simulink model "Copy_of_VTOLTiltrotor"  (R2024a)
settings: configuration reference "VTOLConfiguration" (kept outside this file)
undefined symbols (not defined in the file): airspeed, Battery, BCE12, BCE_Set_init, BMS_Controller_State, C, Cell10_P, Cell11_P, Cell12_P, Cell1_N, Cell1_P, Cell2_P, Cell3_P, Cell4_P, Cell5_P, Cell6_P, Cell7_P, Cell8_P, Cell9_P, Cell_Temperatures, Cell_Voltages, Charging_State, CityMission, control, controlParams, ControlSampleTime, CriticalTiltAngle, currentFactor, CV_Gain, ddx, ddy, ddz, Device_01, DiscIntNeverNeededParam, dx, dy, dz, Earth, env, F, F28379D_ADC_MaxCount, F28379D_ADC_Vmax, FixedWingMission, flightState, Foc_Ki_IxTcpu, Foc_Ki_S, Foc_Kp_I, Foc_Kp_S, fractalcoef, FSState, FWControlParams, HoverMission, I_cc, Ia_offset, Ib_offset, iniRoll, initPitch, iniYaw, IO334, IO334_DAC_Vmax ... (+55)
libraries: slrealtimeethercatlib x109, simulink x81, fl_lib x65, slpidlib x49, mcbcontrolslib x48, nesl_utility x43, speedgoatlib_hdlCoder_IO3xx x31, canmsglib x17, slrealtimeutilitieslib x13, mcbhdlplantlib x13, speedgoatlib_IO611 x12, dspstat3 x12
(part 11 of 20)

== system Copy_of_VTOLTiltrotor/Flight Controller/Autopilot/Multicopter Controller/Horizontal Position Control/XY Controller ==
  X_ref : Inport
  Y_ref : Inport  Port=2
  States : Inport  Port=3
  Bus Selector : BusSelector  OutputSignals=Xe,Ve,Euler
  Demux : Demux  Outputs=3
  Demux1 : Demux  Outputs=3
  Demux2 : Demux  Outputs=3
  Gain : Gain
  Saturation : Saturate  UpperLimit=5  LowerLimit=-5
  Saturation1 : Saturate  UpperLimit=5  LowerLimit=-5
  Sum{,1..3} (4 alike) : Sum  Inputs=|+-
  Terminator{,1..3} (4 alike) : Terminator
  Vx Controller : slpidlib/PID Controller  Controller=P  Form=Parallel  TimeDomain=Discrete-time  UseExternalTs=off  SampleTime=0.005  IntegratorMethod=Forward Euler  FilterMethod=Forward Euler  ControllerParametersSource=internal  P=controlParams.P_VX  I=0  UseKiTs=off  D=0.0379422021775223  UseExternalDerivativeSource=off  N=1.96946409823213  UseFilter=on  TunerSelectOption=Transfer Function Based (PID Tuner App)  InitialConditionSource=internal  InitialConditionForIntegrator=0  InitialConditionForFilter=0  DifferentiatorICPrevScaledInput=0  ExternalReset=none  TrackingMode=off  Kt=1  LimitOutput=off  SatLimitsSource=internal  UpperSaturationLimit=inf  LowerSaturationLimit=-inf  LinearizeAsGain=on  AntiWindupMode=none  Kb=1  LimitIntegrator=off  UpperIntegratorSaturationLimit=inf  LowerIntegratorSaturationLimit=-inf  POutMin=[]  POutMax=[]  IOutMin=[]  IOutMax=[]  DOutMin=[]  DOutMax=[]  NOutMin=[]  NOutMax=[]  SumOutMin=[]  SumOutMax=[]  SaturationOutMin=[]  SaturationOutMax=[]  PParamMin=[]  PParamMax=[]  IParamMin=[]  IParamMax=[]  DParamMin=[]  DParamMax=[]  NParamMin=[]  NParamMax=[]  KbParamMin=[]  KbParamMax=[]  KtParamMin=[]  KtParamMax=[]  KbOutMin=[]  KbOutMax=[]  KtOutMin=[]  KtOutMax=[]  IntegratorOutMin=[]  IntegratorOutMax=[]  FilterOutMin=[]  FilterOutMax=[]  SumI1OutMin=[]  SumI1OutMax=[]  SumI2OutMin=[]  SumI2OutMax=[]  SumI3OutMin=[]  SumI3OutMax=[]  SumI4OutMin=[]  SumI4OutMax=[]  SumDOutMin=[]  SumDOutMax=[]  DifferentiatorOutMin=[]  DifferentiatorOutMax=[]  FilterDiffOutCoefMin=[]  FilterDiffOutCoefMax=[]  ReciprocalOutMin=[]  ReciprocalOutMax=[]  SumDenOutMin=[]  SumDenOutMax=[]  SumNumOutMin=[]  SumNumOutMax=[]  DivideOutMin=[]  DivideOutMax=[]  UdiffTsProdOutMin=[]  UdiffTsProdOutMax=[]  NTsProdOutMin=[]  NTsProdOutMax=[]  UintegralTsProdOutMin=[]  UintegralTsProdOutMax=[]  UngainTsProdOutMin=[]  UngainTsProdOutMax=[]  ClampingZeroOutDataTypeStr=Inherit: Inherit via back propagation  ClampingZeroOutMin=[]  ClampingZeroOutMax=[]  FilterDenConstantOutDataTypeStr=Inherit: Inherit via back propagation  FilterDenConstantOutMin=[]  FilterDenConstantOutMax=[]  PCopyOutDataTypeStr=Inherit: Inherit via back propagation  PCopyOutMin=[]  PCopyOutMax=[]  NCopyOutDataTypeStr=Inherit: Inherit via back propagation  NCopyOutMin=[]  NCopyOutMax=[]  IntegratorContinuousStateAttributes=''  IntegratorStateMustResolveToSignalObject=off  IntegratorRTWStateStorageClass=Auto  FilterContinuousStateAttributes=''  FilterStateMustResolveToSignalObject=off  FilterRTWStateStorageClass=Auto  ParallelPVariant=InternalParameters  IdealPVariant=Disabled  IVariant=Disabled  DVariant=Disabled  IntegratorVariant=Disabled  SatVariant=Disabled  AWVariant=Disabled  PCopyVariant=Disabled  TRVariant=Disabled  FdbkBlocksVariant=Forward  IdealPFdbkVariant=Disabled  SatFdbkVariant=Disabled  DerivativeFilterVariant=Disabled  NVariant=Disabled  NCopyVariant=Disabled_SignalSpec  FilterICVariant=Disabled  IntegratorICVariant=Disabled  ExternalResetVariant=Disabled  TRSumVariant=Passthrough  SumFdbkVariant=Disabled  SumVariant=Passthrough_P  TsampFilterVariant=InternalTs  TsampNgainVariant=Passthrough  TsampIntegralVariant=Disabled_SignalSpec  ExternalSaturationOutDataTypeStr=Inherit: Same as second input  DerivativeSourceVariant=Disabled
  Vy Controller : slpidlib/PID Controller  Controller=P  Form=Parallel  TimeDomain=Discrete-time  UseExternalTs=off  SampleTime=0.005  IntegratorMethod=Forward Euler  FilterMethod=Forward Euler  ControllerParametersSource=internal  P=controlParams.P_VY  I=0  UseKiTs=off  D=0.0379422021775223  UseExternalDerivativeSource=off  N=1.96946409823213  UseFilter=on  TunerSelectOption=Transfer Function Based (PID Tuner App)  InitialConditionSource=internal  InitialConditionForIntegrator=0  InitialConditionForFilter=0  DifferentiatorICPrevScaledInput=0  ExternalReset=none  TrackingMode=off  Kt=1  LimitOutput=off  SatLimitsSource=internal  UpperSaturationLimit=inf  LowerSaturationLimit=-inf  LinearizeAsGain=on  AntiWindupMode=none  Kb=1  LimitIntegrator=off  UpperIntegratorSaturationLimit=inf  LowerIntegratorSaturationLimit=-inf  RndMeth=Round  POutMin=[]  POutMax=[]  IOutMin=[]  IOutMax=[]  DOutMin=[]  DOutMax=[]  NOutMin=[]  NOutMax=[]  SumOutMin=[]  SumOutMax=[]  SaturationOutMin=[]  SaturationOutMax=[]  PParamMin=[]  PParamMax=[]  IParamMin=[]  IParamMax=[]  DParamMin=[]  DParamMax=[]  NParamMin=[]  NParamMax=[]  KbParamMin=[]  KbParamMax=[]  KtParamMin=[]  KtParamMax=[]  KbOutMin=[]  KbOutMax=[]  KtOutMin=[]  KtOutMax=[]  IntegratorOutMin=[]  IntegratorOutMax=[]  FilterOutMin=[]  FilterOutMax=[]  SumI1OutMin=[]  SumI1OutMax=[]  SumI2OutMin=[]  SumI2OutMax=[]  SumI3OutMin=[]  SumI3OutMax=[]  SumI4OutMin=[]  SumI4OutMax=[]  SumDOutMin=[]  SumDOutMax=[]  DifferentiatorOutMin=[]  DifferentiatorOutMax=[]  FilterDiffOutCoefMin=[]  FilterDiffOutCoefMax=[]  ReciprocalOutMin=[]  ReciprocalOutMax=[]  SumDenOutMin=[]  SumDenOutMax=[]  SumNumOutMin=[]  SumNumOutMax=[]  DivideOutMin=[]  DivideOutMax=[]  UdiffTsProdOutMin=[]  UdiffTsProdOutMax=[]  NTsProdOutMin=[]  NTsProdOutMax=[]  UintegralTsProdOutMin=[]  UintegralTsProdOutMax=[]  UngainTsProdOutMin=[]  UngainTsProdOutMax=[]  ClampingZeroOutDataTypeStr=Inherit: Inherit via back propagation  ClampingZeroOutMin=[]  ClampingZeroOutMax=[]  FilterDenConstantOutDataTypeStr=Inherit: Inherit via back propagation  FilterDenConstantOutMin=[]  FilterDenConstantOutMax=[]  PCopyOutDataTypeStr=Inherit: Inherit via back propagation  PCopyOutMin=[]  PCopyOutMax=[]  NCopyOutDataTypeStr=Inherit: Inherit via back propagation  NCopyOutMin=[]  NCopyOutMax=[]  IntegratorContinuousStateAttributes=''  IntegratorStateMustResolveToSignalObject=off  IntegratorRTWStateStorageClass=Auto  FilterContinuousStateAttributes=''  FilterStateMustResolveToSignalObject=off  FilterRTWStateStorageClass=Auto  ParallelPVariant=InternalParameters  IdealPVariant=Disabled  IVariant=Disabled  DVariant=Disabled  IntegratorVariant=Disabled  SatVariant=Disabled  AWVariant=Disabled  PCopyVariant=Disabled  TRVariant=Disabled  FdbkBlocksVariant=Forward  IdealPFdbkVariant=Disabled  SatFdbkVariant=Disabled  DerivativeFilterVariant=Disabled  NVariant=Disabled  NCopyVariant=Disabled_SignalSpec  FilterICVariant=Disabled  IntegratorICVariant=Disabled  ExternalResetVariant=Disabled  TRSumVariant=Passthrough  SumFdbkVariant=Disabled  SumVariant=Passthrough_P  TsampFilterVariant=InternalTs  TsampNgainVariant=Passthrough  TsampIntegralVariant=Disabled_SignalSpec  ExternalSaturationOutDataTypeStr=Inherit: Same as second input  DerivativeSourceVariant=Disabled
  X Controller : slpidlib/PID Controller  Controller=PID  Form=Parallel  TimeDomain=Discrete-time  UseExternalTs=off  SampleTime=-1  IntegratorMethod=Forward Euler  FilterMethod=Forward Euler  ControllerParametersSource=internal  P=controlParams.P_X  I=controlParams.I_X  UseKiTs=off  D=controlParams.D_X  UseExternalDerivativeSource=off  N=controlParams.N_X  UseFilter=on  TunerSelectOption=Transfer Function Based (PID Tuner App)  InitialConditionSource=internal  InitialConditionForIntegrator=0  InitialConditionForFilter=0  DifferentiatorICPrevScaledInput=0  ExternalReset=none  TrackingMode=off  Kt=1  LimitOutput=off  SatLimitsSource=internal  UpperSaturationLimit=inf  LowerSaturationLimit=-inf  LinearizeAsGain=on  AntiWindupMode=none  Kb=1  LimitIntegrator=off  UpperIntegratorSaturationLimit=inf  LowerIntegratorSaturationLimit=-inf  POutMin=[]  POutMax=[]  IOutMin=[]  IOutMax=[]  DOutMin=[]  DOutMax=[]  NOutMin=[]  NOutMax=[]  SumOutMin=[]  SumOutMax=[]  SaturationOutMin=[]  SaturationOutMax=[]  PParamMin=[]  PParamMax=[]  IParamMin=[]  IParamMax=[]  DParamMin=[]  DParamMax=[]  NParamMin=[]  NParamMax=[]  KbParamMin=[]  KbParamMax=[]  KtParamMin=[]  KtParamMax=[]  KbOutMin=[]  KbOutMax=[]  KtOutMin=[]  KtOutMax=[]  IntegratorOutMin=[]  IntegratorOutMax=[]  FilterOutMin=[]  FilterOutMax=[]  SumI1OutMin=[]  SumI1OutMax=[]  SumI2OutMin=[]  SumI2OutMax=[]  SumI3OutMin=[]  SumI3OutMax=[]  SumI4OutMin=[]  SumI4OutMax=[]  SumDOutMin=[]  SumDOutMax=[]  DifferentiatorOutMin=[]  DifferentiatorOutMax=[]  FilterDiffOutCoefMin=[]  FilterDiffOutCoefMax=[]  ReciprocalOutMin=[]  ReciprocalOutMax=[]  SumDenOutMin=[]  SumDenOutMax=[]  SumNumOutMin=[]  SumNumOutMax=[]  DivideOutMin=[]  DivideOutMax=[]  UdiffTsProdOutMin=[]  UdiffTsProdOutMax=[]  NTsProdOutMin=[]  NTsProdOutMax=[]  UintegralTsProdOutMin=[]  UintegralTsProdOutMax=[]  UngainTsProdOutMin=[]  UngainTsProdOutMax=[]  ClampingZeroOutDataTypeStr=Inherit: Inherit via back propagation  ClampingZeroOutMin=[]  ClampingZeroOutMax=[]  FilterDenConstantOutDataTypeStr=Inherit: Inherit via back propagation  FilterDenConstantOutMin=[]  FilterDenConstantOutMax=[]  PCopyOutDataTypeStr=Inherit: Inherit via back propagation  PCopyOutMin=[]  PCopyOutMax=[]  NCopyOutDataTypeStr=Inherit: Inherit via back propagation  NCopyOutMin=[]  NCopyOutMax=[]  IntegratorContinuousStateAttributes=''  IntegratorStateMustResolveToSignalObject=off  IntegratorRTWStateStorageClass=Auto  FilterContinuousStateAttributes=''  FilterStateMustResolveToSignalObject=off  FilterRTWStateStorageClass=Auto  ParallelPVariant=InternalParameters  IdealPVariant=Disabled  IVariant=InternalParameters  DVariant=InternalParameters  IntegratorVariant=Discrete  SatVariant=Disabled  AWVariant=Passthrough  PCopyVariant=Disabled  TRVariant=Disabled  FdbkBlocksVariant=Forward  IdealPFdbkVariant=Disabled  SatFdbkVariant=Disabled  DerivativeFilterVariant=ForwardEulerFilter  NVariant=InternalParameters  NCopyVariant=Disabled  FilterICVariant=InternalICsFilter  IntegratorICVariant=InternalICs  ExternalResetVariant=Disabled  TRSumVariant=Passthrough  SumFdbkVariant=Disabled  SumVariant=Sum_PID  TsampFilterVariant=InternalTs  TsampNgainVariant=Passthrough  TsampIntegralVariant=Disabled_SignalSpec  ExternalSaturationOutDataTypeStr=Inherit: Same as second input  DerivativeSourceVariant=ErrorSignal
  Y Controller : slpidlib/PID Controller  Controller=PI  Form=Parallel  TimeDomain=Discrete-time  UseExternalTs=off  SampleTime=-1  IntegratorMethod=Forward Euler  FilterMethod=Forward Euler  ControllerParametersSource=internal  P=controlParams.P_Y  I=controlParams.I_Y  UseKiTs=off  D=controlParams.D_Y/10  UseExternalDerivativeSource=off  N=controlParams.N_Y  UseFilter=on  TunerSelectOption=Transfer Function Based (PID Tuner App)  InitialConditionSource=internal  InitialConditionForIntegrator=0  InitialConditionForFilter=0  DifferentiatorICPrevScaledInput=0  ExternalReset=none  TrackingMode=off  Kt=1  LimitOutput=off  SatLimitsSource=internal  UpperSaturationLimit=0.4  LowerSaturationLimit=-0.4  LinearizeAsGain=on  AntiWindupMode=clamping  Kb=1  LimitIntegrator=off  UpperIntegratorSaturationLimit=inf  LowerIntegratorSaturationLimit=-inf  POutMin=[]  POutMax=[]  IOutMin=[]  IOutMax=[]  DOutMin=[]  DOutMax=[]  NOutMin=[]  NOutMax=[]  SumOutMin=[]  SumOutMax=[]  SaturationOutMin=[]  SaturationOutMax=[]  PParamMin=[]  PParamMax=[]  IParamMin=[]  IParamMax=[]  DParamMin=[]  DParamMax=[]  NParamMin=[]  NParamMax=[]  KbParamMin=[]  KbParamMax=[]  KtParamMin=[]  KtParamMax=[]  KbOutMin=[]  KbOutMax=[]  KtOutMin=[]  KtOutMax=[]  IntegratorOutMin=[]  IntegratorOutMax=[]  FilterOutMin=[]  FilterOutMax=[]  SumI1OutMin=[]  SumI1OutMax=[]  SumI2OutMin=[]  SumI2OutMax=[]  SumI3OutMin=[]  SumI3OutMax=[]  SumI4OutMin=[]  SumI4OutMax=[]  SumDOutMin=[]  SumDOutMax=[]  DifferentiatorOutMin=[]  DifferentiatorOutMax=[]  FilterDiffOutCoefMin=[]  FilterDiffOutCoefMax=[]  ReciprocalOutMin=[]  ReciprocalOutMax=[]  SumDenOutMin=[]  SumDenOutMax=[]  SumNumOutMin=[]  SumNumOutMax=[]  DivideOutMin=[]  DivideOutMax=[]  UdiffTsProdOutMin=[]  UdiffTsProdOutMax=[]  NTsProdOutMin=[]  NTsProdOutMax=[]  UintegralTsProdOutMin=[]  UintegralTsProdOutMax=[]  UngainTsProdOutMin=[]  UngainTsProdOutMax=[]  ClampingZeroOutDataTypeStr=Inherit: Inherit via back propagation  ClampingZeroOutMin=[]  ClampingZeroOutMax=[]  FilterDenConstantOutDataTypeStr=Inherit: Inherit via back propagation  FilterDenConstantOutMin=[]  FilterDenConstantOutMax=[]  PCopyOutDataTypeStr=Inherit: Inherit via back propagation  PCopyOutMin=[]  PCopyOutMax=[]  NCopyOutDataTypeStr=Inherit: Inherit via back propagation  NCopyOutMin=[]  NCopyOutMax=[]  IntegratorContinuousStateAttributes=''  IntegratorStateMustResolveToSignalObject=off  IntegratorRTWStateStorageClass=Auto  FilterContinuousStateAttributes=''  FilterStateMustResolveToSignalObject=off  FilterRTWStateStorageClass=Auto  ParallelPVariant=InternalParameters  IdealPVariant=Disabled  IVariant=InternalParameters  DVariant=Disabled  IntegratorVariant=Discrete  SatVariant=Disabled  AWVariant=Passthrough  PCopyVariant=Disabled  TRVariant=Disabled  FdbkBlocksVariant=Forward  IdealPFdbkVariant=Disabled  SatFdbkVariant=Disabled  DerivativeFilterVariant=Disabled  NVariant=Disabled  NCopyVariant=Disabled_SignalSpec  FilterICVariant=Disabled  IntegratorICVariant=InternalICs  ExternalResetVariant=Disabled  TRSumVariant=Passthrough  SumFdbkVariant=Disabled  SumVariant=Sum_PI  TsampFilterVariant=InternalTs  TsampNgainVariant=Passthrough  TsampIntegralVariant=Disabled_SignalSpec  ExternalSaturationOutDataTypeStr=Inherit: Same as second input  DerivativeSourceVariant=Disabled
  Yaw Correction : MATLAB Function  TreatAsAtomicUnit=on
  Forward cmd : Outport
  Sideward Cmd : Outport  Port=2
  wires:
  Sum/1 -> X Controller/1
  Demux/3 -> Terminator/1
  Demux2/3 -> Yaw Correction/3(yaw)
  Yaw Correction/1(ucmd) -> Forward cmd/1
  Bus Selector/3 -> Demux2/1  "<Euler>"
  Demux1/1 -> Sum2/2
  Demux/1 -> Sum/2
  Demux/2 -> Sum1/2
  Demux2/2 -> Terminator3/1
  Demux2/1 -> Terminator2/1
  Sum1/1 -> Y Controller/1
  Sum2/1 -> Vx Controller/1
  Yaw Correction/2(vcmd) -> Sideward Cmd/1
  Demux1/3 -> Terminator1/1
  States/1 -> Bus Selector/1
  Bus Selector/1 -> Demux/1  "<Xe>"
  Bus Selector/2 -> Demux1/1  "<Ve>"
  Vx Controller/1 -> Yaw Correction/1(xcmd)
  Demux1/2 -> Gain/1
  Sum3/1 -> Vy Controller/1
  Gain/1 -> Sum3/2
  Vy Controller/1 -> Yaw Correction/2(ycmd)
  Saturation/1 -> Sum3/1
  Saturation1/1 -> Sum2/1
  Y_ref/1 -> Sum1/1
  X_ref/1 -> Sum/1
  X Controller/1 -> Saturation1/1
  Y Controller/1 -> Saturation/1

== system Copy_of_VTOLTiltrotor/Flight Controller/Autopilot/Multicopter Controller/Subsystem/Triggered Subsystem ==
  YawHold : Inport
  Trigger : TriggerPort  VariantControl=(inherit)
  Reference : Outport
  wires:
  YawHold/1 -> Reference/1

== system Copy_of_VTOLTiltrotor/Flight Controller/Guidance Test Bench/ControlType/Guidance Testbench/Control Rate Transition ==
  "1 " : Inport
  In2 : Inport  Port=2
  In3 : Inport  Port=3
  In4 : Inport  Port=4
  In5 : Inport  Port=5
  Rate Transition{,1..3} (4 alike) : RateTransition  OutPortSampleTime=ControlSampleTime
  Rate Transition4 : RateTransition  InitialCondition=flightState.Hover  OutPortSampleTime=ControlSampleTime
  Out1 : Outport
  Out2 : Outport  Port=2
  Out3 : Outport  Port=3
  Out4 : Outport  Port=4
  Out5 : Outport  Port=5
  wires:
  In4/1 -> Rate Transition3/1
  In2/1 -> Rate Transition1/1
  Rate Transition4/1 -> Out5/1
  In5/1 -> Rate Transition4/1
  Rate Transition3/1 -> Out4/1
  "1 "/1 -> Rate Transition/1
  Rate Transition1/1 -> Out2/1
  In3/1 -> Rate Transition2/1
  Rate Transition2/1 -> Out3/1
  Rate Transition/1 -> Out1/1

== system Copy_of_VTOLTiltrotor/Flight Controller/Guidance Test Bench/ControlType/Guidance Testbench/Guidance Logic ==
  UAVState : Inport
  GCSCommands : Inport  Port=2
  Atan2 : Trigonometry  Operator=atan2
  Bus Creator : BusCreator  Inputs=4
  Bus Selector1 : BusSelector  OutputSignals=x,y,z,vy,vx
  Demux : Demux
  Guidance Stateflow : Subsystem
  Interface : Subsystem
  Mux : Mux
  Mux2 : Mux  Inputs=2
  Subsystem : Subsystem
  HoverGuidance : Outport
  FixedWingSP : Outport  Port=2
  AACSP : Outport  Port=3
  ctrlMode : Outport  Port=4
  FlightMode : Outport  Port=5
  wires:
  Mux/1 -> Guidance Stateflow/1(Pose)
  Bus Selector1/5 -> Atan2/2  "<vx>"
  GCSCommands/1 -> Guidance Stateflow/2(GCSCommands)
  Bus Selector1/4 -> Atan2/1  "<vy>"
  Bus Selector1/3 -> Mux2/2, Mux/3  "<z>"
  Bus Selector1/2 -> Mux/2  "<y>"
  UAVState/1 -> Subsystem/1(UAVState), Interface/1(UAVState)
  Bus Selector1/1 -> Mux/1  "<x>"
  Guidance Stateflow/1(HoverCommands) -> Demux/1
  Interface/1(States) -> Bus Selector1/1
  Demux/3 -> Bus Creator/3  "Z"
  Demux/1 -> Bus Creator/1  "X"
  Demux/2 -> Bus Creator/2  "Y"
  Mux2/1 -> Guidance Stateflow/3(LandingStates)
  Atan2/1 -> Mux2/1, Mux/4
  Subsystem/1(States) -> Guidance Stateflow/4(States)
  Guidance Stateflow/3(FixedWingSP) -> FixedWingSP/1
  Guidance Stateflow/2(AACSP) -> AACSP/1
  Guidance Stateflow/4(ctrlMode) -> ctrlMode/1
  Guidance Stateflow/5(FlightMode) -> FlightMode/1
  Bus Creator/1 -> HoverGuidance/1
  Demux/4 -> Bus Creator/4  "Yaw"

== system Copy_of_VTOLTiltrotor/Flight Controller/Guidance Test Bench/ControlType/Manual Control/Command Interface ==
  note: Limit rate for Manual control to keep Flight in operational envelope
  Global Mission : Inport
  Aircraft States : Inport  Port=2
  Airspeed : Constant  Value=16
  Altitude : Constant  Value=1.781376518218607
  Basic Control  Switching : Stateflow chart  TreatAsAtomicUnit=on
  Bus Creator : BusCreator  Inputs=5  OutDataTypeStr=Bus: AAC
  Bus Creator1 : BusCreator  Inputs=4  OutDataTypeStr=Bus: FixedWingCommandBus
  Bus Creator2 : BusCreator  Inputs=4
  Constant{,1..2,5..6} (5 alike) : Constant  Value=0
  Constant4 : Constant  Value=25
  Control Rate Transition : Subsystem
  Course : Constant  Value=0
  Data Type Conversion : DataTypeConversion  OutDataTypeStr=Enum: flightState  SaturateOnIntegerOverflow=off  RndMeth=Floor
  Degrees to Radians : simulink_extras/Transformations/Degrees to Radians
  FlightModeSlider : Constant  Value=0  OutDataTypeStr=uint8
  Gain : Gain  Gain=-1
  Rate Limiter : RateLimiter  RisingSlewLimit=3  FallingSlewLimit=-3  SampleTimeMode=inherited
  Subsystem : Subsystem
  Terminator1 : Terminator
  X : Constant  Value=30
  Y : Constant  Value=30
  Z : Constant  Value=50
  ctrlMode : Outport
  FixedWingSP : Outport  Port=2
  AACSP : Outport  Port=3
  PositionCmds : Outport  Port=4
  FlightMode : Outport  Port=5
  wires:
  Global Mission/1 -> Terminator1/1
  Altitude/1 -> Bus Creator/2  "altitude"
  Bus Creator2/1 -> Control Rate Transition/5(Position)
  Constant5/1 -> Bus Creator/5  "climbrate"
  Course/1 -> Degrees to Radians/1
  Bus Creator/1 -> Control Rate Transition/4(AACSetpoint)
  Z/1 -> Gain/1  "Z"
  Data Type Conversion/1 -> Control Rate Transition/1(FM), Basic Control  Switching/1(FlightMode)
  Constant/1 -> Bus Creator1/1  "roll"
  Bus Creator1/1 -> Control Rate Transition/3(FixedWingSetpoint)
  Constant1/1 -> Bus Creator1/2  "pitch"
  Constant4/1 -> Bus Creator/4  "L1"
  Constant2/1 -> Bus Creator1/3  "yaw"
  Airspeed/1 -> Bus Creator1/4, Bus Creator/1  "airspeed"
  Control Rate Transition/2(FixedWingSP) -> FixedWingSP/1
  Degrees to Radians/1 -> Bus Creator/3  "course"
  X/1 -> Bus Creator2/1  "X"
  Aircraft States/1 -> Subsystem/1(UAVState)
  Y/1 -> Bus Creator2/2  "Y"
  Gain/1 -> Rate Limiter/1  "Z"
  Basic Control  Switching/1(controlMode) -> Control Rate Transition/2("ControlMode ")
  Control Rate Transition/1(ctrlMode) -> ctrlMode/1
  Control Rate Transition/3(AACSP) -> AACSP/1
  Control Rate Transition/4(PositionCmds) -> PositionCmds/1
  Control Rate Transition/5(FlightMode) -> FlightMode/1
  FlightModeSlider/1 -> Data Type Conversion/1
  Subsystem/1(States) -> Basic Control  Switching/2(States)
  Constant6/1 -> Bus Creator2/4
  Rate Limiter/1 -> Bus Creator2/3  "Z"

== system Copy_of_VTOLTiltrotor/Motor Control/Controller/Controller_MIL/F28379D Firmware/Controller Algorithm ==
  Ia_PU : Inport
  QEP_Position_Count : Inport  Port=2
  QEP_Index_Latch : Inport  Port=3
  SpdCmd : Inport  Port=4
  Kp_S : Inport  Port=5
  Ki_S : Inport  Port=6
  EnClosedLoop : Inport  Port=7
  EnablePWM : Inport  Port=8
  Kp_i : Inport  Port=9
  Ki_ixTcpu : Inport  Port=10
  AND : Logic  IconShape=distinctive  AllPortsSameDT=off  OutDataTypeStr=boolean
  Data Type Conversion : DataTypeConversion  OutDataTypeStr=single  SaturateOnIntegerOverflow=off  RndMeth=Floor
  Demux : Demux  Outputs=2
  FOC : Subsystem
  Gain : Gain  Gain=PU_System_I_base
  Gain1 : Gain  Gain=PU_System_N_base
  Mux : Mux  Inputs=2
  Speed and Pos Decoder : Subsystem
  pmsm.PositionOffset : Constant  Value=0  SampleTime=-1
  ModWave : Outport
  PWM_Enable : Outport  Port=2
  fbk_CAN : Outport  Port=3
  wires:
  EnClosedLoop/1 -> AND/2
  Speed and Pos Decoder/1(Theta_e) -> FOC/2(Pos)
  Ia_PU/1 -> FOC/1(Iab), Gain/1
  EnablePWM/1 -> FOC/6(EnablePWM)
  Speed and Pos Decoder/3(IndexFound) -> AND/1
  AND/1 -> FOC/4(EnClosedLoop)
  pmsm.PositionOffset/1 -> Speed and Pos Decoder/3(Offset)
  Speed and Pos Decoder/2(speed) -> FOC/3(Speedfb), Gain1/1
  FOC/2(PWM_Enable) -> PWM_Enable/1
  QEP_Index_Latch/1 -> Speed and Pos Decoder/2(QEP_Index_Latch)
  FOC/1(ModWave) -> ModWave/1  "ModWave"
  Kp_S/1 -> FOC/7(Kp_S)
  Ki_S/1 -> FOC/8(Ki_S)
  SpdCmd/1 -> FOC/5(SpeedRef)
  [Speed] -> Mux/1
  [Pos] -> Mux/2
  Mux/1 -> fbk_CAN/1
  Demux/1 -> [Ia_PU]
  Demux/2 -> [Ib_PU]
  Kp_i/1 -> FOC/9(Kp_i)
  Ki_ixTcpu/1 -> FOC/10(Ki_ixTcpu)
  Gain/1 -> Demux/1
  Gain1/1 -> [Speed]
  QEP_Position_Count/1 -> Speed and Pos Decoder/1(QEP_Position_Count), Data Type Conversion/1
  Data Type Conversion/1 -> [Pos]

== system Copy_of_VTOLTiltrotor/Motor Control/Controller/Controller_MIL/F28379D Firmware/Phase_Current_Rescaling ==
  Ia_ADC : Inport
  Ib_ADC : Inport  Port=2
  IaOffset : Inport  Port=3
  IbOffset : Inport  Port=4
  ADCtoA : Gain  Gain=10/IO334_DAC_Vmax/IO334_iDAC_gain  RndMeth=Simplest  OutDataTypeStr=Inherit: Same as input
  Add : Sum  Inputs=+-
  Add Constant : Bias  Bias=-2^11*IO334_DAC_Vmax/F28379D_ADC_Vmax  SaturateOnIntegerOverflow=off
  Get ADC Voltage : Gain  Gain=F28379D_ADC_Vmax/F28379D_ADC_MaxCount  OutDataTypeStr=single  RndMeth=Simplest
  Mux : Mux  Inputs=2
  Mux1 : Mux  Inputs=2
  PU_Conversion : Gain  Gain=1/PU_System_I_base  RndMeth=Simplest  OutDataTypeStr=Inherit: Same as input
  Rate Transition : RateTransition
  Iab_meas_PU : Outport  VectorParamsAs1DForOutWhenUnconnected=off
  wires:
  Mux1/1 -> Rate Transition/1
  Ia_ADC/1 -> Mux/1
  Ib_ADC/1 -> Mux/2
  Mux/1 -> Add Constant/1
  PU_Conversion/1 -> Iab_meas_PU/1
  IaOffset/1 -> Mux1/1
  IbOffset/1 -> Mux1/2
  Add Constant/1 -> Get ADC Voltage/1
  Get ADC Voltage/1 -> ADCtoA/1  "Currents_inDACvoltages"
  Rate Transition/1 -> Add/2
  ADCtoA/1 -> Add/1  "Currents_A"
  Add/1 -> PU_Conversion/1  "Currents_no_offset"

== system Copy_of_VTOLTiltrotor/Motor Control/Controller/Controller_MIL/F28379D Firmware/Speed Conditioning ==
  Spd[rpm] : Inport
  hz2pu : Gain  Gain=60/(PU_System_N_base *Maxon_645604_Np)  RndMeth=Simplest  OutDataTypeStr=Inherit: Same as input
  rads2hz : Gain  Gain=Maxon_645604_Np/(2*pi)
  rmp2rads : Gain  Gain=2*pi/60
  Spd[PU] : Outport
  wires:
  Spd[rpm]/1 -> rmp2rads/1
  rmp2rads/1 -> rads2hz/1
  rads2hz/1 -> hz2pu/1
  hz2pu/1 -> Spd[PU]/1

== system Copy_of_VTOLTiltrotor/Motor Control/Controller1/Controller_MIL/F28379D Firmware/Controller Algorithm ==
  Ia_PU : Inport
  QEP_Position_Count : Inport  Port=2
  QEP_Index_Latch : Inport  Port=3
  SpdCmd : Inport  Port=4
  Kp_S : Inport  Port=5
  Ki_S : Inport  Port=6
  EnClosedLoop : Inport  Port=7
  EnablePWM : Inport  Port=8
  Kp_i : Inport  Port=9
  Ki_ixTcpu : Inport  Port=10
  AND : Logic  IconShape=distinctive  AllPortsSameDT=off  OutDataTypeStr=boolean
  Data Type Conversion : DataTypeConversion  OutDataTypeStr=single  SaturateOnIntegerOverflow=off  RndMeth=Floor
  Demux : Demux  Outputs=2
  FOC : Subsystem
  Gain : Gain  Gain=PU_System_I_base
  Gain1 : Gain  Gain=PU_System_N_base
  Mux : Mux  Inputs=2
  Speed and Pos Decoder : Subsystem
  pmsm.PositionOffset : Constant  Value=0  SampleTime=-1
  ModWave : Outport
  PWM_Enable : Outport  Port=2
  fbk_CAN : Outport  Port=3
  wires:
  EnClosedLoop/1 -> AND/2
  Speed and Pos Decoder/1(Theta_e) -> FOC/2(Pos)
  Ia_PU/1 -> FOC/1(Iab), Gain/1
  EnablePWM/1 -> FOC/6(EnablePWM)
  Speed and Pos Decoder/3(IndexFound) -> AND/1
  AND/1 -> FOC/4(EnClosedLoop)
  pmsm.PositionOffset/1 -> Speed and Pos Decoder/3(Offset)
  Speed and Pos Decoder/2(speed) -> FOC/3(Speedfb), Gain1/1
  FOC/2(PWM_Enable) -> PWM_Enable/1
  QEP_Index_Latch/1 -> Speed and Pos Decoder/2(QEP_Index_Latch)
  FOC/1(ModWave) -> ModWave/1  "ModWave"
  Kp_S/1 -> FOC/7(Kp_S)
  Ki_S/1 -> FOC/8(Ki_S)
  SpdCmd/1 -> FOC/5(SpeedRef)
  [Speed] -> Mux/1
  [Pos] -> Mux/2
  Mux/1 -> fbk_CAN/1
  Demux/1 -> [Ia_PU]
  Demux/2 -> [Ib_PU]
  Kp_i/1 -> FOC/9(Kp_i)
  Ki_ixTcpu/1 -> FOC/10(Ki_ixTcpu)
  Gain/1 -> Demux/1
  Gain1/1 -> [Speed]
  QEP_Position_Count/1 -> Speed and Pos Decoder/1(QEP_Position_Count), Data Type Conversion/1
  Data Type Conversion/1 -> [Pos]

== system Copy_of_VTOLTiltrotor/Motor Control/Controller1/Controller_MIL/F28379D Firmware/Phase_Current_Rescaling ==
  Ia_ADC : Inport
  Ib_ADC : Inport  Port=2
  IaOffset : Inport  Port=3
  IbOffset : Inport  Port=4
  ADCtoA : Gain  Gain=10/IO334_DAC_Vmax/IO334_iDAC_gain  RndMeth=Simplest  OutDataTypeStr=Inherit: Same as input
  Add : Sum  Inputs=+-
  Add Constant : Bias  Bias=-2^11*IO334_DAC_Vmax/F28379D_ADC_Vmax  SaturateOnIntegerOverflow=off
  Get ADC Voltage : Gain  Gain=F28379D_ADC_Vmax/F28379D_ADC_MaxCount  OutDataTypeStr=single  RndMeth=Simplest
  Mux : Mux  Inputs=2
  Mux1 : Mux  Inputs=2
  PU_Conversion : Gain  Gain=1/PU_System_I_base  RndMeth=Simplest  OutDataTypeStr=Inherit: Same as input
  Rate Transition : RateTransition
  Iab_meas_PU : Outport  VectorParamsAs1DForOutWhenUnconnected=off
  wires:
  Mux1/1 -> Rate Transition/1
  Ia_ADC/1 -> Mux/1
  Ib_ADC/1 -> Mux/2
  Mux/1 -> Add Constant/1
  PU_Conversion/1 -> Iab_meas_PU/1
  IaOffset/1 -> Mux1/1
  IbOffset/1 -> Mux1/2
  Add Constant/1 -> Get ADC Voltage/1
  Get ADC Voltage/1 -> ADCtoA/1  "Currents_inDACvoltages"
  Rate Transition/1 -> Add/2
  ADCtoA/1 -> Add/1  "Currents_A"
  Add/1 -> PU_Conversion/1  "Currents_no_offset"

== system Copy_of_VTOLTiltrotor/Motor Control/Controller1/Controller_MIL/F28379D Firmware/Speed Conditioning ==
  Spd[rpm] : Inport
  hz2pu : Gain  Gain=60/(PU_System_N_base *Maxon_645604_Np)  RndMeth=Simplest  OutDataTypeStr=Inherit: Same as input
  rads2hz : Gain  Gain=Maxon_645604_Np/(2*pi)
  rmp2rads : Gain  Gain=2*pi/60
  Spd[PU] : Outport
  wires:
  Spd[rpm]/1 -> rmp2rads/1
  rmp2rads/1 -> rads2hz/1
  rads2hz/1 -> hz2pu/1
  hz2pu/1 -> Spd[PU]/1

== system Copy_of_VTOLTiltrotor/Motor Control/Controller2/Controller_MIL/F28379D Firmware/Controller Algorithm ==
  Ia_PU : Inport
  QEP_Position_Count : Inport  Port=2
  QEP_Index_Latch : Inport  Port=3
  SpdCmd : Inport  Port=4
  Kp_S : Inport  Port=5
  Ki_S : Inport  Port=6
  EnClosedLoop : Inport  Port=7
  EnablePWM : Inport  Port=8
  Kp_i : Inport  Port=9
  Ki_ixTcpu : Inport  Port=10
  AND : Logic  IconShape=distinctive  AllPortsSameDT=off  OutDataTypeStr=boolean
  Data Type Conversion : DataTypeConversion  OutDataTypeStr=single  SaturateOnIntegerOverflow=off  RndMeth=Floor
  Demux : Demux  Outputs=2
  FOC : Subsystem
  Gain : Gain  Gain=PU_System_I_base
  Gain1 : Gain  Gain=PU_System_N_base
  Mux : Mux  Inputs=2
  Speed and Pos Decoder : Subsystem
  pmsm.PositionOffset : Constant  Value=0  SampleTime=-1
  ModWave : Outport
  PWM_Enable : Outport  Port=2
  fbk_CAN : Outport  Port=3
  wires:
  EnClosedLoop/1 -> AND/2
  Speed and Pos Decoder/1(Theta_e) -> FOC/2(Pos)
  Ia_PU/1 -> FOC/1(Iab), Gain/1
  EnablePWM/1 -> FOC/6(EnablePWM)
  Speed and Pos Decoder/3(IndexFound) -> AND/1
  AND/1 -> FOC/4(EnClosedLoop)
  pmsm.PositionOffset/1 -> Speed and Pos Decoder/3(Offset)
  Speed and Pos Decoder/2(speed) -> FOC/3(Speedfb), Gain1/1
  FOC/2(PWM_Enable) -> PWM_Enable/1
  QEP_Index_Latch/1 -> Speed and Pos Decoder/2(QEP_Index_Latch)
  FOC/1(ModWave) -> ModWave/1  "ModWave"
  Kp_S/1 -> FOC/7(Kp_S)
  Ki_S/1 -> FOC/8(Ki_S)
  SpdCmd/1 -> FOC/5(SpeedRef)
  [Speed] -> Mux/1
  [Pos] -> Mux/2
  Mux/1 -> fbk_CAN/1
  Demux/1 -> [Ia_PU]
  Demux/2 -> [Ib_PU]
  Kp_i/1 -> FOC/9(Kp_i)
  Ki_ixTcpu/1 -> FOC/10(Ki_ixTcpu)
  Gain/1 -> Demux/1
  Gain1/1 -> [Speed]
  QEP_Position_Count/1 -> Speed and Pos Decoder/1(QEP_Position_Count), Data Type Conversion/1
  Data Type Conversion/1 -> [Pos]

== system Copy_of_VTOLTiltrotor/Motor Control/Controller2/Controller_MIL/F28379D Firmware/Phase_Current_Rescaling ==
  Ia_ADC : Inport
  Ib_ADC : Inport  Port=2
  IaOffset : Inport  Port=3
  IbOffset : Inport  Port=4
  ADCtoA : Gain  Gain=10/IO334_DAC_Vmax/IO334_iDAC_gain  RndMeth=Simplest  OutDataTypeStr=Inherit: Same as input
  Add : Sum  Inputs=+-
  Add Constant : Bias  Bias=-2^11*IO334_DAC_Vmax/F28379D_ADC_Vmax  SaturateOnIntegerOverflow=off
  Get ADC Voltage : Gain  Gain=F28379D_ADC_Vmax/F28379D_ADC_MaxCount  OutDataTypeStr=single  RndMeth=Simplest
  Mux : Mux  Inputs=2
  Mux1 : Mux  Inputs=2
  PU_Conversion : Gain  Gain=1/PU_System_I_base  RndMeth=Simplest  OutDataTypeStr=Inherit: Same as input
  Rate Transition : RateTransition
  Iab_meas_PU : Outport  VectorParamsAs1DForOutWhenUnconnected=off
  wires:
  Mux1/1 -> Rate Transition/1
  Ia_ADC/1 -> Mux/1
  Ib_ADC/1 -> Mux/2
  Mux/1 -> Add Constant/1
  PU_Conversion/1 -> Iab_meas_PU/1
  IaOffset/1 -> Mux1/1
  IbOffset/1 -> Mux1/2
  Add Constant/1 -> Get ADC Voltage/1
  Get ADC Voltage/1 -> ADCtoA/1  "Currents_inDACvoltages"
  Rate Transition/1 -> Add/2
  ADCtoA/1 -> Add/1  "Currents_A"
  Add/1 -> PU_Conversion/1  "Currents_no_offset"

== system Copy_of_VTOLTiltrotor/Motor Control/Controller2/Controller_MIL/F28379D Firmware/Speed Conditioning ==
  Spd[rpm] : Inport
  hz2pu : Gain  Gain=60/(PU_System_N_base *Maxon_645604_Np)  RndMeth=Simplest  OutDataTypeStr=Inherit: Same as input
  rads2hz : Gain  Gain=Maxon_645604_Np/(2*pi)
  rmp2rads : Gain  Gain=2*pi/60
  Spd[PU] : Outport
  wires:
  Spd[rpm]/1 -> rmp2rads/1
  rmp2rads/1 -> rads2hz/1
  rads2hz/1 -> hz2pu/1
  hz2pu/1 -> Spd[PU]/1

== system Copy_of_VTOLTiltrotor/Motor Control/Controller3/Controller_MIL/F28379D Firmware/Controller Algorithm ==
  Ia_PU : Inport
  QEP_Position_Count : Inport  Port=2
  QEP_Index_Latch : Inport  Port=3
  SpdCmd : Inport  Port=4
  Kp_S : Inport  Port=5
  Ki_S : Inport  Port=6
  EnClosedLoop : Inport  Port=7
  EnablePWM : Inport  Port=8
  Kp_i : Inport  Port=9
  Ki_ixTcpu : Inport  Port=10
  AND : Logic  IconShape=distinctive  AllPortsSameDT=off  OutDataTypeStr=boolean
  Data Type Conversion : DataTypeConversion  OutDataTypeStr=single  SaturateOnIntegerOverflow=off  RndMeth=Floor
  Demux : Demux  Outputs=2
  FOC : Subsystem
  Gain : Gain  Gain=PU_System_I_base
  Gain1 : Gain  Gain=PU_System_N_base
  Mux : Mux  Inputs=2
  Speed and Pos Decoder : Subsystem
  pmsm.PositionOffset : Constant  Value=0  SampleTime=-1
  ModWave : Outport
  PWM_Enable : Outport  Port=2
  fbk_CAN : Outport  Port=3
  wires:
  EnClosedLoop/1 -> AND/2
  Speed and Pos Decoder/1(Theta_e) -> FOC/2(Pos)
  Ia_PU/1 -> FOC/1(Iab), Gain/1
  EnablePWM/1 -> FOC/6(EnablePWM)
  Speed and Pos Decoder/3(IndexFound) -> AND/1
  AND/1 -> FOC/4(EnClosedLoop)
  pmsm.PositionOffset/1 -> Speed and Pos Decoder/3(Offset)
  Speed and Pos Decoder/2(speed) -> FOC/3(Speedfb), Gain1/1
  FOC/2(PWM_Enable) -> PWM_Enable/1
  QEP_Index_Latch/1 -> Speed and Pos Decoder/2(QEP_Index_Latch)
  FOC/1(ModWave) -> ModWave/1  "ModWave"
  Kp_S/1 -> FOC/7(Kp_S)
  Ki_S/1 -> FOC/8(Ki_S)
  SpdCmd/1 -> FOC/5(SpeedRef)
  [Speed] -> Mux/1
  [Pos] -> Mux/2
  Mux/1 -> fbk_CAN/1
  Demux/1 -> [Ia_PU]
  Demux/2 -> [Ib_PU]
  Kp_i/1 -> FOC/9(Kp_i)
  Ki_ixTcpu/1 -> FOC/10(Ki_ixTcpu)
  Gain/1 -> Demux/1
  Gain1/1 -> [Speed]
  QEP_Position_Count/1 -> Speed and Pos Decoder/1(QEP_Position_Count), Data Type Conversion/1
  Data Type Conversion/1 -> [Pos]

== system Copy_of_VTOLTiltrotor/Motor Control/Controller3/Controller_MIL/F28379D Firmware/Phase_Current_Rescaling ==
  Ia_ADC : Inport
  Ib_ADC : Inport  Port=2
  IaOffset : Inport  Port=3
  IbOffset : Inport  Port=4
  ADCtoA : Gain  Gain=10/IO334_DAC_Vmax/IO334_iDAC_gain  RndMeth=Simplest  OutDataTypeStr=Inherit: Same as input
  Add : Sum  Inputs=+-
  Add Constant : Bias  Bias=-2^11*IO334_DAC_Vmax/F28379D_ADC_Vmax  SaturateOnIntegerOverflow=off
  Get ADC Voltage : Gain  Gain=F28379D_ADC_Vmax/F28379D_ADC_MaxCount  OutDataTypeStr=single  RndMeth=Simplest
  Mux : Mux  Inputs=2
  Mux1 : Mux  Inputs=2
  PU_Conversion : Gain  Gain=1/PU_System_I_base  RndMeth=Simplest  OutDataTypeStr=Inherit: Same as input
  Rate Transition : RateTransition
  Iab_meas_PU : Outport  VectorParamsAs1DForOutWhenUnconnected=off
  wires:
  Mux1/1 -> Rate Transition/1
  Ia_ADC/1 -> Mux/1
  Ib_ADC/1 -> Mux/2
  Mux/1 -> Add Constant/1
  PU_Conversion/1 -> Iab_meas_PU/1
  IaOffset/1 -> Mux1/1
  IbOffset/1 -> Mux1/2
  Add Constant/1 -> Get ADC Voltage/1
  Get ADC Voltage/1 -> ADCtoA/1  "Currents_inDACvoltages"
  Rate Transition/1 -> Add/2
  ADCtoA/1 -> Add/1  "Currents_A"
  Add/1 -> PU_Conversion/1  "Currents_no_offset"

== system Copy_of_VTOLTiltrotor/Motor Control/Controller3/Controller_MIL/F28379D Firmware/Speed Conditioning ==
  Spd[rpm] : Inport
  hz2pu : Gain  Gain=60/(PU_System_N_base *Maxon_645604_Np)  RndMeth=Simplest  OutDataTypeStr=Inherit: Same as input
  rads2hz : Gain  Gain=Maxon_645604_Np/(2*pi)
  rmp2rads : Gain  Gain=2*pi/60
  Spd[PU] : Outport
  wires:
  Spd[rpm]/1 -> rmp2rads/1
  rmp2rads/1 -> rads2hz/1
  rads2hz/1 -> hz2pu/1
  hz2pu/1 -> Spd[PU]/1

== system Copy_of_VTOLTiltrotor/Motor Control/Three-Phase PMSM Drive/PMSM and average inverter/Encoder Simulation/Get_PU  ==
  rad : Inport
  Constant2 : Constant  Value=2*pi  OutDataTypeStr=single  SampleTime=-1
  Get_PU : Gain  Gain=1/(2*pi)  RndMeth=Simplest  OutDataTypeStr=Inherit: Same as input
  Mod : Math  Operator=mod
  PU : Outport  VectorParamsAs1DForOutWhenUnconnected=off
  wires:
  Get_PU/1 -> PU/1
  Mod/1 -> Get_PU/1
  Constant2/1 -> Mod/2
  rad/1 -> Mod/1

== system Copy_of_VTOLTiltrotor/Motor Control/Three-Phase PMSM Drive/PMSM and average inverter/Encoder Simulation/Wrap ==
  in : Inport
  Constant2 : Constant  OutDataTypeStr=single  SampleTime=-1
  Mod : Math  Operator=mod
  out : Outport  VectorParamsAs1DForOutWhenUnconnected=off
  wires:
  Mod/1 -> out/1
  Constant2/1 -> Mod/2
  in/1 -> Mod/1

== system Copy_of_VTOLTiltrotor/Motor Control/Three-Phase PMSM Drive/PMSM and average inverter/Runtime to DC/To Dc A1 ==
  A_on : Inport
  A_off : Inport  Port=2
  Add : Sum
  Add Constant1 : Bias  Bias=1  SaturateOnIntegerOverflow=off
  Data Type Conversion3 : DataTypeConversion  OutDataTypeStr=double  SaturateOnIntegerOverflow=off  RndMeth=Floor
  Data Type Conversion5 : DataTypeConversion  OutDataTypeStr=double  SaturateOnIntegerOverflow=off  RndMeth=Floor
  Divide : Product  Inputs=*/
  Gain1 : Gain  Gain=-2
  Dc : Outport
  wires:
  Data Type Conversion5/1 -> Add/2
  Add Constant1/1 -> Dc/1
  Gain1/1 -> Add Constant1/1
  Add/1 -> Divide/2
  Data Type Conversion3/1 -> Add/1, Divide/1
  A_off/1 -> Data Type Conversion5/1
  Divide/1 -> Gain1/1
  A_on/1 -> Data Type Conversion3/1

== system Copy_of_VTOLTiltrotor/Motor Control/Three-Phase PMSM Drive/PMSM and average inverter/Runtime to DC/To Dc A2 ==
  A_on : Inport
  A_off : Inport  Port=2
  Add : Sum
  Add Constant1 : Bias  Bias=1  SaturateOnIntegerOverflow=off
  Data Type Conversion3 : DataTypeConversion  OutDataTypeStr=double  SaturateOnIntegerOverflow=off  RndMeth=Floor
  Data Type Conversion5 : DataTypeConversion  OutDataTypeStr=double  SaturateOnIntegerOverflow=off  RndMeth=Floor
  Divide : Product  Inputs=*/
  Gain1 : Gain  Gain=-2
  Dc : Outport
  wires:
  A_on/1 -> Data Type Conversion3/1
  Divide/1 -> Gain1/1
  A_off/1 -> Data Type Conversion5/1
  Data Type Conversion3/1 -> Divide/1, Add/1
  Add/1 -> Divide/2
  Gain1/1 -> Add Constant1/1
  Add Constant1/1 -> Dc/1
  Data Type Conversion5/1 -> Add/2

== system Copy_of_VTOLTiltrotor/Motor Control/Three-Phase PMSM Drive/PMSM and average inverter/Runtime to DC/To Dc A3 ==
  A_on : Inport
  A_off : Inport  Port=2
  Add : Sum
  Add Constant1 : Bias  Bias=1  SaturateOnIntegerOverflow=off
  Data Type Conversion3 : DataTypeConversion  OutDataTypeStr=double  SaturateOnIntegerOverflow=off  RndMeth=Floor
  Data Type Conversion5 : DataTypeConversion  OutDataTypeStr=double  SaturateOnIntegerOverflow=off  RndMeth=Floor
  Divide : Product  Inputs=*/
  Gain1 : Gain  Gain=-2
  Dc : Outport
  wires:
  Data Type Conversion5/1 -> Add/2
  Add Constant1/1 -> Dc/1
  Gain1/1 -> Add Constant1/1
  Add/1 -> Divide/2
  Data Type Conversion3/1 -> Add/1, Divide/1
  A_off/1 -> Data Type Conversion5/1
  Divide/1 -> Gain1/1
  A_on/1 -> Data Type Conversion3/1

== system Copy_of_VTOLTiltrotor/Motor Control/Three-Phase PMSM Drive/PMSM and inverter with switching dynamics/DAC Config/Subsystem ==
  Plant_frequency : Inport
  SignalFrequency : Inport  Port=2
  Add : Sum  Inputs=+-
  Data Type Conversion : DataTypeConversion  OutDataTypeStr=uint16  SaturateOnIntegerOverflow=off  RndMeth=Floor
  Divide : Product  Inputs=*/
  constant : Constant  VectorParams1D=off  SampleTime=-1
  DAC_reset : Outport
  wires:
  SignalFrequency/1 -> Divide/2
  Add/1 -> Data Type Conversion/1
  Divide/1 -> Add/1
  Data Type Conversion/1 -> DAC_reset/1
  constant/1 -> Add/2
  Plant_frequency/1 -> Divide/1

== system Copy_of_VTOLTiltrotor/Motor Control/Three-Phase PMSM Drive/PMSM and inverter with switching dynamics/Encoder Simulation/Get_PU  ==
  rad : Inport
  Constant2 : Constant  Value=2*pi  OutDataTypeStr=single  SampleTime=-1
  Get_PU : Gain  Gain=1/(2*pi)  RndMeth=Simplest  OutDataTypeStr=Inherit: Same as input
  Mod : Math  Operator=mod
  PU : Outport  VectorParamsAs1DForOutWhenUnconnected=off
  wires:
  Get_PU/1 -> PU/1
  Mod/1 -> Get_PU/1
  Constant2/1 -> Mod/2
  rad/1 -> Mod/1

== system Copy_of_VTOLTiltrotor/Motor Control/Three-Phase PMSM Drive/PMSM and inverter with switching dynamics/Encoder Simulation/Wrap ==
  in : Inport
  Constant2 : Constant  OutDataTypeStr=single  SampleTime=-1
  Mod : Math  Operator=mod
  out : Outport  VectorParamsAs1DForOutWhenUnconnected=off
  wires:
  Mod/1 -> out/1
  Constant2/1 -> Mod/2
  in/1 -> Mod/1
